simulink model "TrailerSoftware"  (R2019b)
settings: Solver=FixedStepDiscrete  StartTime=0.0  StopTime=inf  FixedStep=update  RelTol=1e-3  EnableMultiTasking=on
values from neighbouring files (symbols this model uses):
  countmax1 = 2500    [ProductionMfile.m]
  countmax2 = 2500    [ProductionMfile.m]
  HeaterIntGain = .0008    (= 0.0008)    [ProductionMfile.m]
  HeatGain = 10    [ProductionMfile.m]
  Intll = 0    [ProductionMfile.m]
  MaxCondPressure = 350    [ProductionMfile.m]
  MinSP = 1    [ProductionMfile.m]
  PostGain100 = 0.0002    [ProductionMfile.m]
  PostGain150 = 0.0005    [ProductionMfile.m]
  PostGain200 = 0.0004    [ProductionMfile.m]
  PostGain300 = 0.0008    [ProductionMfile.m]
  PostInit150 = 12    [ProductionMfile.m]
  PostIntulC = 65    [ProductionMfile.m]
  PostPGain = 0    [ProductionMfile.m]
  PreGain100 = 0.0005    [ProductionMfile.m]
  PreGain150 = 0.0005    [ProductionMfile.m]
  PreGain200 = 0.0003    [ProductionMfile.m]
  PreGain300 = 0.0008    [ProductionMfile.m]
  PreInit150 = 30    [ProductionMfile.m]
  PreIntulC = 65    [ProductionMfile.m]
  PreIntulDH = 65    [ProductionMfile.m]
  PrePGain = 0    [ProductionMfile.m]
  SatPress = [10 20 30 40 50 60 70 80 90 100 110 120 130 140 150 160 170      180 190 200 210 220 230 240 250 260 270 280 290 300 310 320 330      340 350 360 370 380 390 400 410 420 430 440 450 460 470 480 490      500]    [ProductionMfile.m]
  SatTemp = [-29.497 -2.4046 15.401 29.047 40.267 49.88 58.338 65.922 72.819      79.159 85.037 90.526 95.68 100.55 105.16 109.54 113.73 117.73 121.57      125.26 128.82 132.25 135.56 138.77 141.88 144.89 147.82 150.67 153.44      156.15 158.78 161.35 163.85 166.3 168.7 171.04 173.33 175.58 177.77      179.93 182.04 184.11 186.14 188.14 190.09 192.01 193.9 195.75 197.58      199.37]    [ProductionMfile.m]
  SHGain = 2    [ProductionMfile.m]
  SizeCANMatrix = 80    [ProductionMfile.m]
  SizeCOBIDVector = 10    [ProductionMfile.m]
  update = 0.002    [ProductionMfile.m]
undefined symbols (not defined in the file or in its folder): DiscIntNeverNeededParam, PostDGain, PreDGain, Ratio100, Ratio150, Ratio200, Ratio300
libraries: simulink x60, c2837xDlib x35, xpcutilitieslib x24, c2802xlib x8, c280xlib x7, etargetslib x4, svdutilitieslib x2, c2000lib x1
(part 4 of 8)

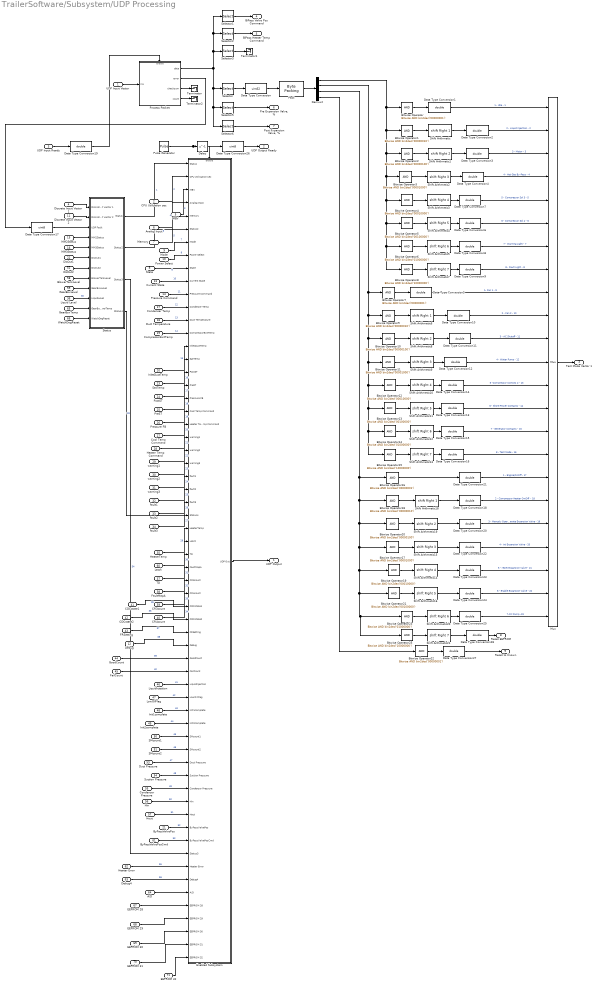
== system TrailerSoftware/Subsystem/UDP Processing ==
  UDP Input Vector : Inport  OutDataTypeStr=uint8  PortDimensions=SizeUDPInput  SampleTime=update  LockScale=on
  CPU Utilization sec : Inport  Port=2  OutDataTypeStr=double  PortDimensions=1  SampleTime=update
  UDP Input Ready : Inport  Port=3  OutDataTypeStr=boolean  PortDimensions=1  SampleTime=update
  Discrete Input Vector 1 : Inport  Port=4  OutDataTypeStr=uint8  PortDimensions=16  SampleTime=update
  MBV : Inport  Port=5  OutDataTypeStr=double  PortDimensions=MBVS  SampleTime=update
  Analog Input : Inport  Port=6
  Memory : Inport  Port=7
  State : Inport  Port=8
  Mode : Inport  Port=9
  Power Select : Inport  Port=10
  Discrete Input Vector 2 : Inport  Port=11  OutDataTypeStr=uint8  PortDimensions=16  SampleTime=update
  Debug : Inport  Port=12  PortDimensions=1
  Current State : Inport  Port=13  PortDimensions=1
  Pressure Command : Inport  Port=14
  MM2Status : Inport  Port=15
  MM3Status : Inport  Port=16  OutDataTypeStr=uint8  PortDimensions=1  SampleTime=update
  Condenser Temp : Inport  Port=17
  Duct Temperature : Inport  Port=18
  CompressorExitTemp : Inport  Port=19
  InletDuctTemp : Inport  Port=20
  ByPassValvePos : Inport  Port=21  OutDataTypeStr=double  SampleTime=update
  DisOut1 : Inport  Port=22  OutDataTypeStr=uint8  SampleTime=update
  SatTemp : Inport  Port=23
  PostST : Inport  Port=24
  PreST : Inport  Port=25
  Pressure FB : Inport  Port=26
  Cool Temp Command : Inport  Port=27
  Heater Temp Command : Inport  Port=28
  warning1 : Inport  Port=29
  warning2 : Inport  Port=30
  warning3 : Inport  Port=31
  fault1 : Inport  Port=32
  fault2 : Inport  Port=33
  fault3 : Inport  Port=34
  HeaterTemp : Inport  Port=35
  Liquid Level : Inport  Port=36
  TD : Inport  Port=37
  FaultMapA : Inport  Port=38
  CR3count : Inport  Port=39
  CR4count : Inport  Port=40
  CDCstate1 : Inport  Port=41
  CDCstate2 : Inport  Port=42
  FRSetting : Inport  Port=43
  GoodCount : Inport  Port=44  PortDimensions=1
  FailCount : Inport  Port=45  PortDimensions=1
  LiquidInjection : Inport  Port=46  PortDimensions=1
  LowOilFlag : Inport  Port=47
  Init1complete : Inport  Port=48  PortDimensions=1
  Init2complete : Inport  Port=49  PortDimensions=1
  SMcount1 : Inport  Port=50  PortDimensions=1
  SMcount2 : Inport  Port=51  PortDimensions=1
  DisOut2 : Inport  Port=52  OutDataTypeStr=uint8  SampleTime=update
  Duct Pressure : Inport  Port=53
  Suction Pressure : Inport  Port=54
  Condensor Pressure : Inport  Port=55
  Hin : Inport  Port=56
  Hout : Inport  Port=57
  BlowerTankLevel : Inport  Port=58
  GearBoxLevel : Inport  Port=59
  Latch : Inport  Port=60
  ByPassValvePosCmd : Inport  Port=61  OutDataTypeStr=double  SampleTime=update
  Heater Error : Inport  Port=62  PortDimensions=1
  Debug4 : Inport  Port=63  PortDimensions=1
  A/D : Inport  Port=64  PortDimensions=8
  GearBoxTemp : Inport  Port=65
  WatchDogReset : Inport  Port=66  OutDataTypeStr=uint8  PortDimensions=1  SampleTime=update
  EEPROM 28 : Inport  Port=67
  EEPROM 29 : Inport  Port=68
  EEPROM 30 : Inport  Port=69
  EEPROM 31 : Inport  Port=70
  EEPROM 32 : Inport  Port=71
  Bitwise Operator{,7,16,22} (4 alike) : simulink/Logic and Bit Operations/Bitwise Operator  logicop=AND  UseBitMask=on  BitMask=bin2dec('00000001')  BitMaskRealWorld=Stored Integer
  Bitwise Operator1 : simulink/Logic and Bit Operations/Bitwise Operator  logicop=AND  UseBitMask=on  BitMask=bin2dec('00000010')  BitMaskRealWorld=Stored Integer
  Bitwise Operator10 : simulink/Logic and Bit Operations/Bitwise Operator  logicop=AND  UseBitMask=on  BitMask=bin2dec('00000100')  BitMaskRealWorld=Stored Integer
  Bitwise Operator11 : simulink/Logic and Bit Operations/Bitwise Operator  logicop=AND  UseBitMask=on  BitMask=bin2dec('00001000')  BitMaskRealWorld=Stored Integer
  Bitwise Operator12 : simulink/Logic and Bit Operations/Bitwise Operator  logicop=AND  UseBitMask=on  BitMask=bin2dec('00010000')  BitMaskRealWorld=Stored Integer
  Bitwise Operator13 : simulink/Logic and Bit Operations/Bitwise Operator  logicop=AND  UseBitMask=on  BitMask=bin2dec('00100000')  BitMaskRealWorld=Stored Integer
  Bitwise Operator14 : simulink/Logic and Bit Operations/Bitwise Operator  logicop=AND  UseBitMask=on  BitMask=bin2dec('01000000')  BitMaskRealWorld=Stored Integer
  Bitwise Operator15 : simulink/Logic and Bit Operations/Bitwise Operator  logicop=AND  UseBitMask=on  BitMask=bin2dec('10000000')  BitMaskRealWorld=Stored Integer
  Bitwise Operator17 : simulink/Logic and Bit Operations/Bitwise Operator  logicop=AND  UseBitMask=on  BitMask=bin2dec('00001000')  BitMaskRealWorld=Stored Integer
  Bitwise Operator18 : simulink/Logic and Bit Operations/Bitwise Operator  logicop=AND  UseBitMask=on  BitMask=bin2dec('00000010')  BitMaskRealWorld=Stored Integer
  Bitwise Operator19 : simulink/Logic and Bit Operations/Bitwise Operator  logicop=AND  UseBitMask=on  BitMask=bin2dec('00010000')  BitMaskRealWorld=Stored Integer
  Bitwise Operator2 : simulink/Logic and Bit Operations/Bitwise Operator  logicop=AND  UseBitMask=on  BitMask=bin2dec('00000100')  BitMaskRealWorld=Stored Integer
  Bitwise Operator20 : simulink/Logic and Bit Operations/Bitwise Operator  logicop=AND  UseBitMask=on  BitMask=bin2dec('00000100')  BitMaskRealWorld=Stored Integer
  Bitwise Operator21 : simulink/Logic and Bit Operations/Bitwise Operator  logicop=AND  UseBitMask=on  BitMask=bin2dec('00100000')  BitMaskRealWorld=Stored Integer
  Bitwise Operator23 : simulink/Logic and Bit Operations/Bitwise Operator  logicop=AND  UseBitMask=on  BitMask=bin2dec('01000000')  BitMaskRealWorld=Stored Integer
  Bitwise Operator25 : simulink/Logic and Bit Operations/Bitwise Operator  logicop=AND  UseBitMask=on  BitMask=bin2dec('10000000')  BitMaskRealWorld=Stored Integer
  Bitwise Operator3 : simulink/Logic and Bit Operations/Bitwise Operator  logicop=AND  UseBitMask=on  BitMask=bin2dec('00001000')  BitMaskRealWorld=Stored Integer
  Bitwise Operator4 : simulink/Logic and Bit Operations/Bitwise Operator  logicop=AND  UseBitMask=on  BitMask=bin2dec('00010000')  BitMaskRealWorld=Stored Integer
  Bitwise Operator5 : simulink/Logic and Bit Operations/Bitwise Operator  logicop=AND  UseBitMask=on  BitMask=bin2dec('00100000')  BitMaskRealWorld=Stored Integer
  Bitwise Operator6 : simulink/Logic and Bit Operations/Bitwise Operator  logicop=AND  UseBitMask=on  BitMask=bin2dec('01000000')  BitMaskRealWorld=Stored Integer
  Bitwise Operator8 : simulink/Logic and Bit Operations/Bitwise Operator  logicop=AND  UseBitMask=on  BitMask=bin2dec('10000000')  BitMaskRealWorld=Stored Integer
  Bitwise Operator9 : simulink/Logic and Bit Operations/Bitwise Operator  logicop=AND  UseBitMask=on  BitMask=bin2dec('00000010')  BitMaskRealWorld=Stored Integer
  Data Type Conversion : DataTypeConversion  OutDataTypeStr=uint32
  Data Type Conversion{1..16,18..25,27..28} (26 alike) : DataTypeConversion  OutDataTypeStr=double
  Data Type Conversion17 : DataTypeConversion  OutDataTypeStr=uint8
  Data Type Conversion26 : DataTypeConversion  OutDataTypeStr=uint8
  Delay : Delay  DelayLength=1  InitialCondition=0
  Demux2 : Demux
  Enabled Subsystem : Subsystem  TreatAsAtomicUnit=on
  Mux : Mux  Inputs=23
  Pack : xpcutilitieslib/Byte Packing   MaskPackedDataType=uint8  MaskUnpackedDataTypes={'uint32'}  MaskAlignment=1
  Process Packet : Subsystem
  Pulse Generator : DiscretePulseGenerator  Period=10  SampleTime=update
  Selector : Selector  InputPortWidth=ndmain  IndexOptions=Index vector (dialog)  Indices=[1]  OutputSizes=1
  Selector1 : Selector  InputPortWidth=ndmain  IndexOptions=Index vector (dialog)  Indices=[2]  OutputSizes=1
  Selector2 : Selector  InputPortWidth=ndmain  IndexOptions=Index vector (dialog)  Indices=[3]  OutputSizes=1
  Selector3 : Selector  InputPortWidth=ndmain  IndexOptions=Index vector (dialog)  Indices=[4]  OutputSizes=1
  Selector5 : Selector  InputPortWidth=ndmain  IndexOptions=Index vector (dialog)  Indices=[6]  OutputSizes=1
  Selector6 : Selector  InputPortWidth=ndmain  IndexOptions=Index vector (dialog)  Indices=[7]  OutputSizes=1
  Shift Arithmetic : ArithShift  BitShiftNumber=1  BitShiftDirection=Right
  Shift Arithmetic1 : ArithShift  BitShiftNumber=2  BitShiftDirection=Right
  Shift Arithmetic10 : ArithShift  BitShiftNumber=4  BitShiftDirection=Right
  Shift Arithmetic11 : ArithShift  BitShiftNumber=5  BitShiftDirection=Right
  Shift Arithmetic12 : ArithShift  BitShiftNumber=6  BitShiftDirection=Right
  Shift Arithmetic13 : ArithShift  BitShiftNumber=7  BitShiftDirection=Right
  Shift Arithmetic14 : ArithShift  BitShiftNumber=4  BitShiftDirection=Right
  Shift Arithmetic15 : ArithShift  BitShiftNumber=3  BitShiftDirection=Right
  Shift Arithmetic16 : ArithShift  BitShiftNumber=5  BitShiftDirection=Right
  Shift Arithmetic18 : ArithShift  BitShiftNumber=1  BitShiftDirection=Right
  Shift Arithmetic19 : ArithShift  BitShiftNumber=2  BitShiftDirection=Right
  Shift Arithmetic2 : ArithShift  BitShiftNumber=3  BitShiftDirection=Right
  Shift Arithmetic20 : ArithShift  BitShiftNumber=6  BitShiftDirection=Right
  Shift Arithmetic21 : ArithShift  BitShiftNumber=7  BitShiftDirection=Right
  Shift Arithmetic3 : ArithShift  BitShiftNumber=4  BitShiftDirection=Right
  Shift Arithmetic4 : ArithShift  BitShiftNumber=5  BitShiftDirection=Right
  Shift Arithmetic5 : ArithShift  BitShiftNumber=6  BitShiftDirection=Right
  Shift Arithmetic6 : ArithShift  BitShiftNumber=1  BitShiftDirection=Right
  Shift Arithmetic7 : ArithShift  BitShiftNumber=7  BitShiftDirection=Right
  Shift Arithmetic8 : ArithShift  BitShiftNumber=2  BitShiftDirection=Right
  Shift Arithmetic9 : ArithShift  BitShiftNumber=3  BitShiftDirection=Right
  Status : Subsystem
  Terminator : Terminator
  Terminator1 : Terminator
  Terminator2 : Terminator
  UDP Output : Outport  OutDataTypeStr=uint8  PortDimensions=376  VectorParamsAs1DForOutWhenUnconnected=off
  UDP Output Ready : Outport  Port=2  OutDataTypeStr=uint8  SampleTime=update  VectorParamsAs1DForOutWhenUnconnected=off  LockScale=on
  Test Mode Vector 1 : Outport  Port=3  VectorParamsAs1DForOutWhenUnconnected=off
  BiPass Valve Pos Command : Outport  Port=4  VectorParamsAs1DForOutWhenUnconnected=off
  BiPass Heater Temp Command : Outport  Port=5  VectorParamsAs1DForOutWhenUnconnected=off
  "Pre Expansion Valve, %" : Outport  Port=6  VectorParamsAs1DForOutWhenUnconnected=off
  "Post Expansion Valve, %" : Outport  Port=7  VectorParamsAs1DForOutWhenUnconnected=off
  Reset EEPROM : Outport  Port=8  VectorParamsAs1DForOutWhenUnconnected=off
  Reset to Known : Outport  Port=9  VectorParamsAs1DForOutWhenUnconnected=off
  wires:
  Process Packet/1(data) -> Selector3/1, Selector1/1, Selector2/1, Selector6/1, Selector5/1, Selector/1
  Process Packet/4(count) -> Terminator2/1
  Process Packet/3(checksum) -> Terminator/1
  UDP Input Vector/1 -> Process Packet/1(In1)
  Bitwise Operator/1 -> Data Type Conversion1/1
  Bitwise Operator1/1 -> Shift Arithmetic/1
  Bitwise Operator2/1 -> Shift Arithmetic1/1
  Bitwise Operator3/1 -> Shift Arithmetic2/1
  Data Type Conversion4/1 -> Mux/4  "4 - Hot Gas By-Pass - 4"
  Bitwise Operator5/1 -> Shift Arithmetic4/1
  Data Type Conversion6/1 -> Mux/6  "6 - Compressor Sol 4 - 6"
  Bitwise Operator4/1 -> Shift Arithmetic3/1
  Data Type Conversion7/1 -> Mux/5  "5 - Compressor Sol 3 - 5"
  Shift Arithmetic/1 -> Data Type Conversion2/1
  Shift Arithmetic1/1 -> Data Type Conversion3/1
  Shift Arithmetic2/1 -> Data Type Conversion4/1
  Shift Arithmetic3/1 -> Data Type Conversion7/1
  Shift Arithmetic4/1 -> Data Type Conversion6/1
  Bitwise Operator6/1 -> Shift Arithmetic5/1
  Data Type Conversion8/1 -> Mux/7  "7 - Warning Light - 7"
  Shift Arithmetic5/1 -> Data Type Conversion8/1
  Bitwise Operator8/1 -> Shift Arithmetic7/1
  Shift Arithmetic7/1 -> Data Type Conversion9/1
  Data Type Conversion9/1 -> Mux/8  "8 - Fault Light - 8"
  Data Type Conversion1/1 -> Mux/1  "1 - Idle - 1"
  Data Type Conversion2/1 -> Mux/2  "2 - Liquid Injection - 2"
  Data Type Conversion3/1 -> Mux/3  "3 - Motor - 3"
  Demux2/1 -> Bitwise Operator/1, Bitwise Operator1/1, Bitwise Operator2/1, Bitwise Operator8/1, Bitwise Operator6/1, Bitwise Operator5/1, Bitwise Operator4/1, Bitwise Operator3/1
  Data Type Conversion/1 -> Pack/1
  Pack/1 -> Demux2/1
  Discrete Input Vector 1/1 -> Status/1(Discrete Input Vector 1)
  Status/1("Status ") -> Enabled Subsystem/1(Status)  "1"
  Bitwise Operator7/1 -> Data Type Conversion5/1
  Bitwise Operator9/1 -> Shift Arithmetic6/1
  Bitwise Operator10/1 -> Shift Arithmetic8/1
  Bitwise Operator11/1 -> Shift Arithmetic9/1
  Data Type Conversion12/1 -> Mux/12  "4 - Water Pump - 12"
  Bitwise Operator13/1 -> Shift Arithmetic11/1
  Data Type Conversion13/1 -> Mux/14  "6 - Shore Power Contacts - 14"
  Bitwise Operator12/1 -> Shift Arithmetic10/1
  Data Type Conversion14/1 -> Mux/13  "5 -Compressor Contcts 2 - 13"
  Shift Arithmetic6/1 -> Data Type Conversion10/1
  Shift Arithmetic8/1 -> Data Type Conversion11/1
  Shift Arithmetic9/1 -> Data Type Conversion12/1
  Shift Arithmetic10/1 -> Data Type Conversion14/1
  Shift Arithmetic11/1 -> Data Type Conversion13/1
  Bitwise Operator14/1 -> Shift Arithmetic12/1
  Data Type Conversion15/1 -> Mux/15  "7 - Generator Contacts - 15"
  Shift Arithmetic12/1 -> Data Type Conversion15/1
  Bitwise Operator15/1 -> Shift Arithmetic13/1
  Shift Arithmetic13/1 -> Data Type Conversion16/1
  Data Type Conversion16/1 -> Mux/16  "8 - Test Mode - 16"
  Data Type Conversion10/1 -> Mux/10  "2 - Fan 2 - 10"
  Data Type Conversion11/1 -> Mux/11  "3 - AC Shutoff - 11"
  Demux2/2 -> Bitwise Operator15/1, Bitwise Operator14/1, Bitwise Operator13/1, Bitwise Operator12/1, Bitwise Operator11/1, Bitwise Operator10/1, Bitwise Operator9/1, Bitwise Operator7/1
  Delay/1 -> Data Type Conversion26/1
  Mux/1 -> Test Mode Vector 1/1
  Data Type Conversion5/1 -> Mux/9  "1- Fan 1 - 9"
  CPU Utilization sec/1 -> Enabled Subsystem/2(CPU Utilization sec)  "2"
  MBV/1 -> Enabled Subsystem/3(MBV)  "3"
  Analog Input/1 -> Enabled Subsystem/4(Analog Input)  "4"
  Memory/1 -> Enabled Subsystem/5(Memory)  "5"
  State/1 -> Enabled Subsystem/9(State)  "9"
  Enabled Subsystem/1(UDP Out) -> UDP Output/1
  Mode/1 -> Enabled Subsystem/7(Mode)  "7"
  Power Select/1 -> Enabled Subsystem/8(Power Select)  "8"
  Discrete Input Vector 2/1 -> Status/2(Discrete Input Vector 2)
  Process Packet/2(error) -> Data Type Conversion17/1
  Data Type Conversion17/1 -> Status/3(UDP Fault)
  Current State/1 -> Enabled Subsystem/10(Current State)  "10"
  Pressure Command/1 -> Enabled Subsystem/11(Pressure Command)  "11"
  Selector5/1 -> "Pre Expansion Valve, %"/1
  Selector6/1 -> "Post Expansion Valve, %"/1
  MM3Status/1 -> Status/5(MM3Status)
  MM2Status/1 -> Status/4(MM2Status)
  Condenser Temp/1 -> Enabled Subsystem/12(Condenser Temp)  "12"
  Duct Temperature/1 -> Enabled Subsystem/13(Duct Temperature)  "13"
  CompressorExitTemp/1 -> Enabled Subsystem/14(CompressorExitTemp)  "14"
  Bitwise Operator16/1 -> Data Type Conversion21/1
  Data Type Conversion20/1 -> Mux/19  "3 - Manualy Opererate Expansion Valve - 19"
  Data Type Conversion21/1 -> Mux/17  "1 - Engine/OnOff - 17"
  Selector1/1 -> BiPass Valve Pos Command/1
  Selector2/1 -> BiPass Heater Temp Command/1
  Selector3/1 -> Terminator1/1
  InletDuctTemp/1 -> Enabled Subsystem/15(InletDuctTemp)  "15"
  ByPassValvePos/1 -> Enabled Subsystem/52(ByPassValvePos)  "52"
  DisOut1/1 -> Status/6(DisOut1)
  SatTemp/1 -> Enabled Subsystem/16(SatTemp)  "16"
  PostST/1 -> Enabled Subsystem/17(PostST)  "17"
  PreST/1 -> Enabled Subsystem/18(PreST)  "18"
  Pressure FB/1 -> Enabled Subsystem/19(Pressure FB)  "19"
  Cool Temp Command/1 -> Enabled Subsystem/20(Cool Temp Command)  "20"
  Heater Temp Command/1 -> Enabled Subsystem/21(Heater Temp Command)  "21"
  warning1/1 -> Enabled Subsystem/22(warning1)  "22"
  warning3/1 -> Enabled Subsystem/24(warning3)  "24"
  warning2/1 -> Enabled Subsystem/23(warning2)  "23"
  fault1/1 -> Enabled Subsystem/25(fault1)  "25"
  fault2/1 -> Enabled Subsystem/26(fault2)  "26"
  fault3/1 -> Enabled Subsystem/27(fault3)  "27"
  HeaterTemp/1 -> Enabled Subsystem/29(HeaterTemp)  "29"
  Latch/1 -> Enabled Subsystem/30(Latch)  "30"
  TD/1 -> Enabled Subsystem/31(TD)  "31"
  FaultMapA/1 -> Enabled Subsystem/32(FaultMapA)  "32"
  CR3count/1 -> Enabled Subsystem/33(CR3count)  "33"
  CR4count/1 -> Enabled Subsystem/34(CR4count)  "34"
  CDCstate1/1 -> Enabled Subsystem/35(CDCstate1)  "35"
  CDCstate2/1 -> Enabled Subsystem/36(CDCstate2)  "36"
  Debug/1 -> Enabled Subsystem/38(Debug)  "38"
  Status/2(Status2) -> Enabled Subsystem/6(Status2)  "6"
  FRSetting/1 -> Enabled Subsystem/37(FRSetting)  "37"
  Shift Arithmetic18/1 -> Data Type Conversion18/1
  Data Type Conversion18/1 -> Mux/18  "2 - Compressor Heater On/Off  - 18"
  GoodCount/1 -> Enabled Subsystem/39(GoodCount)  "39"
  FailCount/1 -> Enabled Subsystem/40(FailCount)  "40"
  LiquidInjection/1 -> Enabled Subsystem/41(LiquidInjection)  "41"
  LowOilFlag/1 -> Enabled Subsystem/42(LowOilFlag)  "42"
  Data Type Conversion22/1 -> Mux/20  "4 - int Expansion Valve - 20"
  Data Type Conversion23/1 -> Mux/21  "5 - reset Expansion Valve - 21"
  SMcount1/1 -> Enabled Subsystem/45(SMcount1)  "45"
  Init2complete/1 -> Enabled Subsystem/44(Init2complete)  "44"
  Init1complete/1 -> Enabled Subsystem/43(Init1complete)  "43"
  SMcount2/1 -> Enabled Subsystem/46(SMcount2)  "46"
  Status/4(Status4) -> Enabled Subsystem/28(Status4)  "28"
  Selector/1 -> Data Type Conversion/1
  Bitwise Operator18/1 -> Shift Arithmetic18/1
  Bitwise Operator20/1 -> Shift Arithmetic19/1
  Shift Arithmetic19/1 -> Data Type Conversion20/1
  Bitwise Operator17/1 -> Shift Arithmetic15/1
  Shift Arithmetic15/1 -> Data Type Conversion22/1
  Bitwise Operator19/1 -> Shift Arithmetic14/1
  Shift Arithmetic14/1 -> Data Type Conversion23/1
  Bitwise Operator21/1 -> Shift Arithmetic16/1
  Shift Arithmetic16/1 -> Data Type Conversion24/1
  Data Type Conversion24/1 -> Mux/22  "6 - Enable Expansion Valve - 22"
  DisOut2/1 -> Status/7(DisOut2)
  Bitwise Operator23/1 -> Shift Arithmetic20/1
  Shift Arithmetic20/1 -> Data Type Conversion25/1
  Data Type Conversion25/1 -> Mux/23  "7-Oil Pump -23"
  Duct Pressure/1 -> Enabled Subsystem/47(Duct Pressure)  "47"
  Suction Pressure/1 -> Enabled Subsystem/48(Suction Pressure)  "48"
  Condensor Pressure/1 -> Enabled Subsystem/49(Condensor Pressure)  "49"
  Hout/1 -> Enabled Subsystem/51(Hout)  "51"
  Hin/1 -> Enabled Subsystem/50(Hin)  "50"
  Data Type Conversion26/1 -> UDP Output Ready/1
  BlowerTankLevel/1 -> Status/8(BlowerTankLevel)
  GearBoxLevel/1 -> Status/9(GearBoxLevel)
  UDP Input Ready/1 -> Data Type Conversion19/1
  Liquid Level/1 -> Status/10(LiquidLevel)  "30"
  Pulse Generator/1 -> Enabled Subsystem/Enable, Delay/1
  Data Type Conversion19/1 -> Process Packet/Enable
  ByPassValvePosCmd/1 -> Enabled Subsystem/53(ByPassValvePosCmd)  "53"
  Status/3(Status3) -> Enabled Subsystem/54(Status3)  "54"
  Heater Error/1 -> Enabled Subsystem/55(Heater Error)  "55"
  Debug4/1 -> Enabled Subsystem/56(Debug4)  "56"
  A/D/1 -> Enabled Subsystem/57(A/D)
  GearBoxTemp/1 -> Status/11(GearBox OverTemp)
  WatchDogReset/1 -> Status/12(WatchDogReset)
  Data Type Conversion27/1 -> Reset to Known/1
  Bitwise Operator22/1 -> Data Type Conversion27/1
  Demux2/4 -> Bitwise Operator22/1
  Shift Arithmetic21/1 -> Data Type Conversion28/1
  Data Type Conversion28/1 -> Reset EEPROM/1
  EEPROM 28/1 -> Enabled Subsystem/58(EEPROM 28)
  EEPROM 29/1 -> Enabled Subsystem/59(EEPROM 29)
  EEPROM 30/1 -> Enabled Subsystem/60(EEPROM 30)
  EEPROM 31/1 -> Enabled Subsystem/61(EEPROM 31)
  EEPROM 32/1 -> Enabled Subsystem/62(EEPROM 32)
  Demux2/3 -> Bitwise Operator16/1, Bitwise Operator18/1, Bitwise Operator25/1, Bitwise Operator23/1, Bitwise Operator21/1, Bitwise Operator19/1, Bitwise Operator17/1, Bitwise Operator20/1
  Bitwise Operator25/1 -> Shift Arithmetic21/1

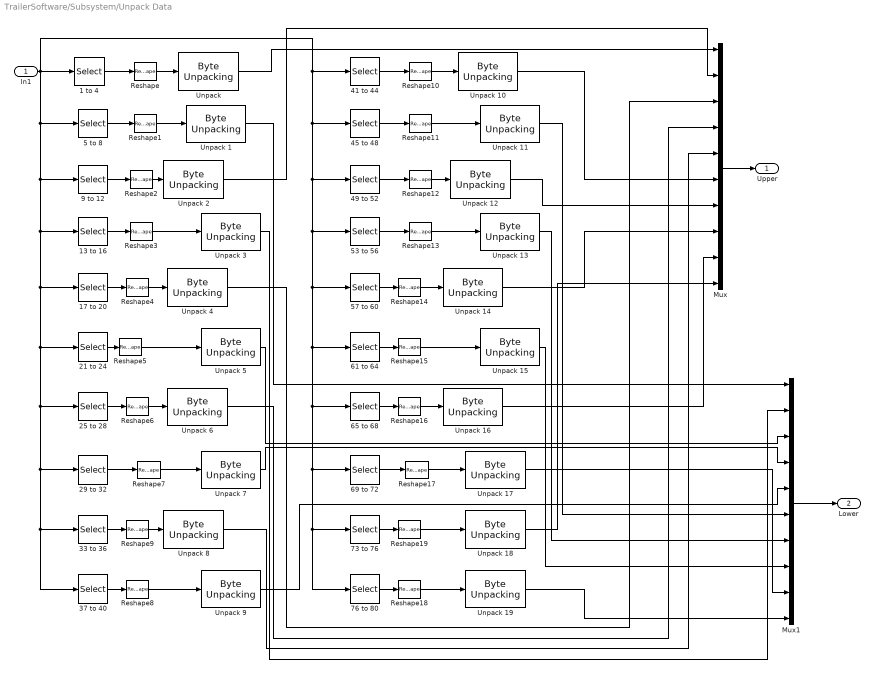
== system TrailerSoftware/Subsystem/Unpack Data ==
  In1 : Inport
  1 to 4 : Selector  InputPortWidth=80  IndexOptions=Index vector (dialog)  Indices=[1:4]  OutputSizes=1
  13 to 16 : Selector  InputPortWidth=80  IndexOptions=Index vector (dialog)  Indices=[13:16]  OutputSizes=1
  17 to 20 : Selector  InputPortWidth=80  IndexOptions=Index vector (dialog)  Indices=[17:20]  OutputSizes=1
  21 to 24 : Selector  InputPortWidth=80  IndexOptions=Index vector (dialog)  Indices=[21:24]  OutputSizes=1
  25 to 28 : Selector  InputPortWidth=80  IndexOptions=Index vector (dialog)  Indices=[25:28]  OutputSizes=1
  29 to 32 : Selector  InputPortWidth=80  IndexOptions=Index vector (dialog)  Indices=[29:32]  OutputSizes=1
  33 to 36 : Selector  InputPortWidth=80  IndexOptions=Index vector (dialog)  Indices=[33:36]  OutputSizes=1
  37 to 40 : Selector  InputPortWidth=80  IndexOptions=Index vector (dialog)  Indices=[37:40]  OutputSizes=1
  41 to 44 : Selector  InputPortWidth=80  IndexOptions=Index vector (dialog)  Indices=[41:44]  OutputSizes=1
  45 to 48 : Selector  InputPortWidth=80  IndexOptions=Index vector (dialog)  Indices=[45:48]  OutputSizes=1
  49 to 52 : Selector  InputPortWidth=80  IndexOptions=Index vector (dialog)  Indices=[49:52]  OutputSizes=1
  5 to 8 : Selector  InputPortWidth=80  IndexOptions=Index vector (dialog)  Indices=[5:8]  OutputSizes=1
  53 to 56 : Selector  InputPortWidth=80  IndexOptions=Index vector (dialog)  Indices=[53:56]  OutputSizes=1
  57 to 60 : Selector  InputPortWidth=80  IndexOptions=Index vector (dialog)  Indices=[57:60]  OutputSizes=1
  61 to 64 : Selector  InputPortWidth=80  IndexOptions=Index vector (dialog)  Indices=[61:64]  OutputSizes=1
  65 to 68 : Selector  InputPortWidth=80  IndexOptions=Index vector (dialog)  Indices=[65:68]  OutputSizes=1
  69 to 72 : Selector  InputPortWidth=80  IndexOptions=Index vector (dialog)  Indices=[69:72]  OutputSizes=1
  73 to 76 : Selector  InputPortWidth=80  IndexOptions=Index vector (dialog)  Indices=[73:76]  OutputSizes=1
  76 to 80 : Selector  InputPortWidth=80  IndexOptions=Index vector (dialog)  Indices=[77:80]  OutputSizes=1
  9 to 12 : Selector  InputPortWidth=80  IndexOptions=Index vector (dialog)  Indices=[9:12]  OutputSizes=1
  Mux : Mux  Inputs=10
  Mux1 : Mux  Inputs=10
  Reshape{,1..19} (20 alike) : Reshape
  Unpack {,1..19} (20 alike) : xpcutilitieslib/Byte Unpacking   MaskUnpackedDataTypes={'uint32'}  MaskUnpackedDataSizes={[1]}  MaskAlignment=1
      settings: SourceProductName=Simulink Real-Time  SourceProductBaseCode=XP
  Upper : Outport  VectorParamsAs1DForOutWhenUnconnected=off
  Lower : Outport  Port=2  VectorParamsAs1DForOutWhenUnconnected=off
  wires:
  1 to 4/1 -> Reshape/1
  5 to 8/1 -> Reshape1/1
  9 to 12/1 -> Reshape2/1
  13 to 16/1 -> Reshape3/1
  17 to 20/1 -> Reshape4/1
  21 to 24/1 -> Reshape5/1
  25 to 28/1 -> Reshape6/1
  29 to 32/1 -> Reshape7/1
  33 to 36/1 -> Reshape9/1
  37 to 40/1 -> Reshape8/1
  41 to 44/1 -> Reshape10/1
  45 to 48/1 -> Reshape11/1
  49 to 52/1 -> Reshape12/1
  53 to 56/1 -> Reshape13/1
  57 to 60/1 -> Reshape14/1
  61 to 64/1 -> Reshape15/1
  65 to 68/1 -> Reshape16/1
  69 to 72/1 -> Reshape17/1
  73 to 76/1 -> Reshape19/1
  76 to 80/1 -> Reshape18/1
  In1/1 -> 37 to 40/1, 33 to 36/1, 29 to 32/1, 25 to 28/1, 21 to 24/1, 17 to 20/1, 13 to 16/1, 9 to 12/1, 5 to 8/1, 76 to 80/1, 73 to 76/1, 69 to 72/1, 65 to 68/1, 61 to 64/1, 57 to 60/1, 53 to 56/1, 49 to 52/1, 45 to 48/1, 41 to 44/1, 1 to 4/1
  "Unpack "/1 -> Mux/1
  Unpack 2/1 -> Mux/2
  Unpack 4/1 -> Mux/3
  Unpack 6/1 -> Mux/4
  Unpack 8/1 -> Mux/5
  Unpack 10/1 -> Mux/6
  Unpack 12/1 -> Mux/7
  Unpack 14/1 -> Mux/8
  Unpack 16/1 -> Mux/9
  Unpack 18/1 -> Mux/10
  Mux/1 -> Upper/1
  Mux1/1 -> Lower/1
  Unpack 1/1 -> Mux1/1
  Unpack 3/1 -> Mux1/2
  Unpack 5/1 -> Mux1/3
  Unpack 7/1 -> Mux1/4
  Unpack 9/1 -> Mux1/5
  Unpack 11/1 -> Mux1/6
  Unpack 13/1 -> Mux1/7
  Unpack 15/1 -> Mux1/8
  Unpack 17/1 -> Mux1/9
  Unpack 19/1 -> Mux1/10
  Reshape/1 -> "Unpack "/1
  Reshape1/1 -> Unpack 1/1
  Reshape2/1 -> Unpack 2/1
  Reshape3/1 -> Unpack 3/1
  Reshape4/1 -> Unpack 4/1
  Reshape5/1 -> Unpack 5/1
  Reshape6/1 -> Unpack 6/1
  Reshape7/1 -> Unpack 7/1
  Reshape8/1 -> Unpack 9/1
  Reshape9/1 -> Unpack 8/1
  Reshape10/1 -> Unpack 10/1
  Reshape11/1 -> Unpack 11/1
  Reshape12/1 -> Unpack 12/1
  Reshape13/1 -> Unpack 13/1
  Reshape14/1 -> Unpack 14/1
  Reshape15/1 -> Unpack 15/1
  Reshape16/1 -> Unpack 16/1
  Reshape17/1 -> Unpack 17/1
  Reshape18/1 -> Unpack 19/1
  Reshape19/1 -> Unpack 18/1

== system TrailerSoftware/Subsystem/Super Heat Control/filter ==
  In1 : Inport
  Discrete-Time Integrator : DiscreteIntegrator  SampleTime=update  ICPrevOutput=DiscIntNeverNeededParam  ICPrevScaledInput=DiscIntNeverNeededParam
  K : Gain  Gain=.25
  Quantizer : Quantizer  QuantizationInterval=.5
  Saturation : Saturate  UpperLimit=3  LowerLimit=-3
  Sum2 : Sum  Inputs=|+-
  Out1 : Outport  VectorParamsAs1DForOutWhenUnconnected=off
  wires:
  Saturation/1 -> Discrete-Time Integrator/1
  In1/1 -> Sum2/1
  Sum2/1 -> K/1
  K/1 -> Saturation/1
  Discrete-Time Integrator/1 -> Sum2/2, Quantizer/1
  Quantizer/1 -> Out1/1

== system TrailerSoftware/Subsystem/Super Heat Control/filter1 ==
  In1 : Inport
  Discrete-Time Integrator : DiscreteIntegrator  SampleTime=update  ICPrevOutput=DiscIntNeverNeededParam  ICPrevScaledInput=DiscIntNeverNeededParam
  K : Gain  Gain=.25
  Quantizer : Quantizer  QuantizationInterval=.5
  Saturation : Saturate  UpperLimit=3  LowerLimit=-3
  Sum2 : Sum  Inputs=|+-
  Out1 : Outport  VectorParamsAs1DForOutWhenUnconnected=off
  wires:
  Saturation/1 -> Discrete-Time Integrator/1
  In1/1 -> Sum2/1
  Sum2/1 -> K/1
  K/1 -> Saturation/1
  Discrete-Time Integrator/1 -> Sum2/2, Quantizer/1
  Quantizer/1 -> Out1/1

== system TrailerSoftware/Subsystem/Super Heat Control/filter2 ==
  In1 : Inport
  Discrete-Time Integrator : DiscreteIntegrator  InitialCondition=70  SampleTime=update  ICPrevOutput=DiscIntNeverNeededParam  ICPrevScaledInput=DiscIntNeverNeededParam
  K : Gain  Gain=.05
  Quantizer : Quantizer  QuantizationInterval=10
  Saturation : Saturate  UpperLimit=3  LowerLimit=-3
  Sum2 : Sum  Inputs=|+-
  Out1 : Outport  VectorParamsAs1DForOutWhenUnconnected=off
  wires:
  Saturation/1 -> Discrete-Time Integrator/1
  In1/1 -> Sum2/1
  Sum2/1 -> K/1
  K/1 -> Saturation/1
  Discrete-Time Integrator/1 -> Sum2/2, Quantizer/1
  Quantizer/1 -> Out1/1

== system TrailerSoftware/Subsystem/Temperature Vector/DegCtoDegF ==
  In1 : Inport
  Constant7 : Constant  Value=32
  Gain9 : Gain  Gain=9/5
  Sum8 : Sum  Inputs=|++
  Out1 : Outport  VectorParamsAs1DForOutWhenUnconnected=off
  wires:
  Sum8/1 -> Out1/1
  In1/1 -> Gain9/1
  Constant7/1 -> Sum8/2
  Gain9/1 -> Sum8/1

== system TrailerSoftware/Subsystem/Temperature Vector/DegCtoDegF1 ==
  In1 : Inport
  Constant7 : Constant  Value=32
  Gain9 : Gain  Gain=9/5
  Sum8 : Sum  Inputs=|++
  Out1 : Outport  VectorParamsAs1DForOutWhenUnconnected=off
  wires:
  Sum8/1 -> Out1/1
  In1/1 -> Gain9/1
  Constant7/1 -> Sum8/2
  Gain9/1 -> Sum8/1

== system TrailerSoftware/Subsystem/Temperature Vector/DegCtoDegF2 ==
  In1 : Inport
  Constant7 : Constant  Value=32
  Gain9 : Gain  Gain=9/5
  Sum8 : Sum  Inputs=|++
  Out1 : Outport  VectorParamsAs1DForOutWhenUnconnected=off
  wires:
  Sum8/1 -> Out1/1
  In1/1 -> Gain9/1
  Constant7/1 -> Sum8/2
  Gain9/1 -> Sum8/1

== system TrailerSoftware/Subsystem/Temperature Vector/DegCtoDegF3 ==
  In1 : Inport
  Constant7 : Constant  Value=32
  Gain9 : Gain  Gain=9/5
  Sum8 : Sum  Inputs=|++
  Out1 : Outport  VectorParamsAs1DForOutWhenUnconnected=off
  wires:
  Sum8/1 -> Out1/1
  In1/1 -> Gain9/1
  Constant7/1 -> Sum8/2
  Gain9/1 -> Sum8/1

== system TrailerSoftware/Subsystem/Temperature Vector/DegCtoDegF4 ==
  In1 : Inport
  Constant7 : Constant  Value=32
  Gain9 : Gain  Gain=9/5
  Sum8 : Sum  Inputs=|++
  Out1 : Outport  VectorParamsAs1DForOutWhenUnconnected=off
  wires:
  Sum8/1 -> Out1/1
  In1/1 -> Gain9/1
  Constant7/1 -> Sum8/2
  Gain9/1 -> Sum8/1

== system TrailerSoftware/Subsystem/Temperature Vector/DegCtoDegF5 ==
  In1 : Inport
  Constant7 : Constant  Value=32
  Gain9 : Gain  Gain=9/5
  Sum8 : Sum  Inputs=|++
  Out1 : Outport  VectorParamsAs1DForOutWhenUnconnected=off
  wires:
  Sum8/1 -> Out1/1
  In1/1 -> Gain9/1
  Constant7/1 -> Sum8/2
  Gain9/1 -> Sum8/1

== system TrailerSoftware/Subsystem/Temperature Vector/DegCtoDegF6 ==
  In1 : Inport
  Constant7 : Constant  Value=32
  Gain9 : Gain  Gain=9/5
  Sum8 : Sum  Inputs=|++
  Out1 : Outport  VectorParamsAs1DForOutWhenUnconnected=off
  wires:
  Sum8/1 -> Out1/1
  In1/1 -> Gain9/1
  Constant7/1 -> Sum8/2
  Gain9/1 -> Sum8/1

== system TrailerSoftware/Subsystem/Temperature Vector/DegCtoDegF7 ==
  In1 : Inport
  Constant7 : Constant  Value=32
  Gain9 : Gain  Gain=9/5
  Sum8 : Sum  Inputs=|++
  Out1 : Outport  VectorParamsAs1DForOutWhenUnconnected=off
  wires:
  Sum8/1 -> Out1/1
  In1/1 -> Gain9/1
  Constant7/1 -> Sum8/2
  Gain9/1 -> Sum8/1

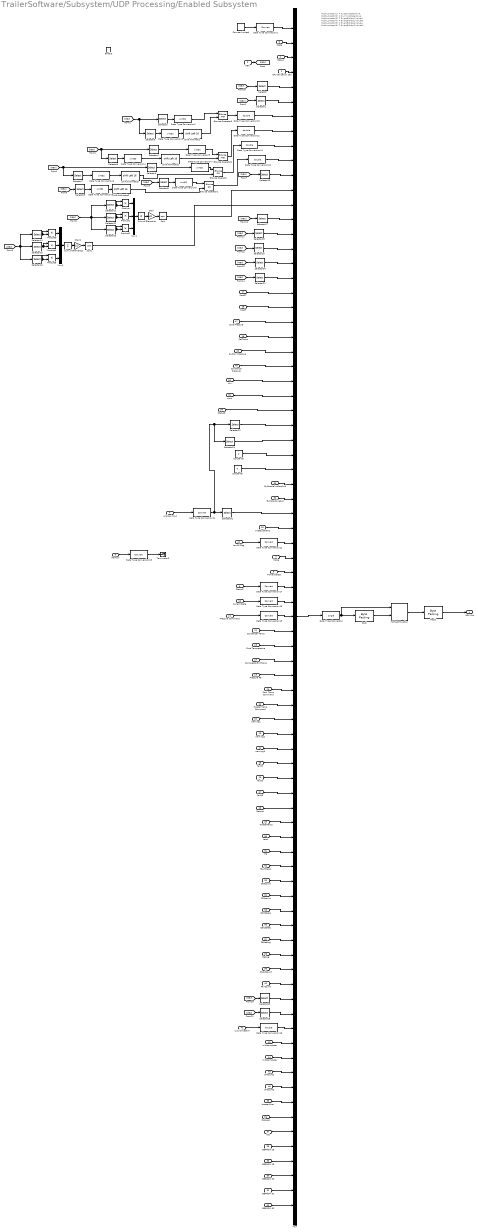
== system TrailerSoftware/Subsystem/UDP Processing/Enabled Subsystem ==
  note: ModbusVector(1) = SystemStateValue;
      | ModbusVector(2) = RunningStateValue;
      | ModbusVector(3) = EventBitMap1ValueA;
      | ModbusVector(4) = EventBitMap1ValueB;
      | ModbusVector(5) = EventBitMap2ValueA;
      | ModbusVector(6) = EventBitMap2ValueB;
      | ModbusVector(7) = FaultBitMapValueA;
      | ModbusVector(8) = FaultBitMapValueB;
      | ModbusVector(9) = WarningBitMapValueA;
      | ModbusVector(10) = WarningBitMapValueB;
      | ModbusVector(11) = GenFreqValue;
      | ModbusVector(12) = GenVoltValueA;
      | ModbusVector(13) = GenVoltValueB;
      | ModbusVector(14) = GenVoltValueC;
      | ModbusVector(15) = GenCurValueA;
      | ModbusVector(16) = GenCurValueB;
      | ModbusVector(17) = GenCurValueC;
      | ModbusVector(18) = EngineTempValue;
      | ModbusVector(19) = EngineOilPressValue;
      | ModbusVector(20) = FuelLevelValue;
      | ModbusVector(21) = BatteryVoltValue;
      | ModbusVector(22) = EngineRunHoursValue;
      | ModbusVector(23) = FCSuperHeatValue;
      | ModbusVector(24) = RCSuperHeatValue;
      | ModbusVector(25) = SuctionPressValue;
      | ModbusVector(26) = FSatTempValue;
      | ModbusVector(27) = RSatTempValue;
      | ModbusVector(28) = FSucTempValue;
      | ModbusVector(29) = RSucTempValue;
      | ModbusVector(30) = FRmTempValue;
      | ModbusVector(31) = RRmTempValue;
      | ModbusVector(32) = FValPosValue;
      | ModbusVector(33) = RValPosValue;
      | ModbusVector(34) = FEvapTempValue;
      | ModbusVector(35) = REvapTempValue;
      | ModbusVector(36) = FAlarmValue;
      | ModbusVector(37) = RAlarmValue;
  Status : Inport
  CPU Utilization sec : Inport  Port=2  OutDataTypeStr=double  PortDimensions=1  SampleTime=update
  MBV : Inport  Port=3  PortDimensions=MBVS
  Analog Input : Inport  Port=4
  Memory : Inport  Port=5
  Status2 : Inport  Port=6
  Mode : Inport  Port=7
  Power Select : Inport  Port=8
  State : Inport  Port=9
  Current State : Inport  Port=10
  Pressure Command : Inport  Port=11
  Condenser Temp : Inport  Port=12
  Duct Temperature : Inport  Port=13
  CompressorExitTemp : Inport  Port=14
  InletDuctTemp : Inport  Port=15
  SatTemp : Inport  Port=16
  PostST : Inport  Port=17
  PreST : Inport  Port=18
  Pressure FB : Inport  Port=19
  Cool Temp Command : Inport  Port=20
  Heater Temp Command : Inport  Port=21
  warning1 : Inport  Port=22
  warning2 : Inport  Port=23
  warning3 : Inport  Port=24
  fault1 : Inport  Port=25
  fault2 : Inport  Port=26
  fault3 : Inport  Port=27
  Status4 : Inport  Port=28
  HeaterTemp : Inport  Port=29
  Latch : Inport  Port=30
  TD : Inport  Port=31
  FaultMapA : Inport  Port=32
  CR3count : Inport  Port=33
  CR4count : Inport  Port=34
  CDCstate1 : Inport  Port=35
  CDCstate2 : Inport  Port=36
  FRSetting : Inport  Port=37
  Debug : Inport  Port=38  PortDimensions=1
  GoodCount : Inport  Port=39  PortDimensions=1
  FailCount : Inport  Port=40  PortDimensions=1
  LiquidInjection : Inport  Port=41  PortDimensions=1
  LowOilFlag : Inport  Port=42
  Init1complete : Inport  Port=43  PortDimensions=1
  Init2complete : Inport  Port=44  PortDimensions=1
  SMcount1 : Inport  Port=45  PortDimensions=1
  SMcount2 : Inport  Port=46  PortDimensions=1
  Duct Pressure : Inport  Port=47
  Suction Pressure : Inport  Port=48
  Condensor Pressure : Inport  Port=49
  Hin : Inport  Port=50
  Hout : Inport  Port=51
  ByPassValvePos : Inport  Port=52  OutDataTypeStr=double  SampleTime=update
  ByPassValvePosCmd : Inport  Port=53  OutDataTypeStr=double  SampleTime=update
  Status3 : Inport  Port=54
  Heater Error : Inport  Port=55  PortDimensions=1
  Debug4 : Inport  Port=56  PortDimensions=1
  A/D : Inport  Port=57  PortDimensions=8
  EEPROM 28 : Inport  Port=58
  EEPROM 29 : Inport  Port=59
  EEPROM 30 : Inport  Port=60
  EEPROM 31 : Inport  Port=61
  EEPROM 32 : Inport  Port=62
  Enable : EnablePort
  Bitwise Operator : simulink/Logic and Bit Operations/Bitwise Operator  logicop=OR  UseBitMask=off  NumInputPorts=2  BitMask=bin2dec('11011001')  BitMaskRealWorld=Stored Integer
  Bitwise Operator1 : simulink/Logic and Bit Operations/Bitwise Operator  logicop=OR  UseBitMask=off  NumInputPorts=2  BitMask=bin2dec('11011001')  BitMaskRealWorld=Stored Integer
  Bitwise Operator2 : simulink/Logic and Bit Operations/Bitwise Operator  logicop=AND  UseBitMask=off  NumInputPorts=2  BitMask=bin2dec('11011001')  BitMaskRealWorld=Stored Integer
  Bitwise Operator3 : simulink/Logic and Bit Operations/Bitwise Operator  logicop=AND  UseBitMask=off  NumInputPorts=2  BitMask=bin2dec('11011001')  BitMaskRealWorld=Stored Integer
  Constant8 : Constant  Value=0
  Constant9 : Constant  Value=0
  Counter Limited : simulink/Sources/Counter Limited  uplimit=2^30  tsamp=-1
  Data Type Conversion : DataTypeConversion  OutDataTypeStr=single
  Data Type Conversion{1,14..15,17..19,21} (7 alike) : DataTypeConversion
  Data Type Conversion{10..13,16} (5 alike) : DataTypeConversion  OutDataTypeStr=double
  Data Type Conversion{2..9} (8 alike) : DataTypeConversion  OutDataTypeStr=uint32
  Gain : Gain  Gain=1/3
  Gain1 : Gain  Gain=1/3
  MATLAB Function : MATLAB Function
  Mux : Mux  Inputs=81
  Mux1 : Mux  Inputs=3
  Mux2 : Mux  Inputs=3
  Pack : xpcutilitieslib/Byte Packing   MaskPackedDataType=uint8  MaskUnpackedDataTypes={'single'}  MaskAlignment=1
  Pack1 : xpcutilitieslib/Byte Packing   MaskPackedDataType=uint8  MaskUnpackedDataTypes={'single'}  MaskAlignment=4
  Product{,1..5} (6 alike) : Product
  Selector : Selector  InputPortWidth=MBVS  IndexOptions=Index vector (dialog)  Indices=[1]  OutputSizes=1
  Selector1 : Selector  InputPortWidth=MBVS  IndexOptions=Index vector (dialog)  Indices=[2]  OutputSizes=1
  Selector10 : Selector  IndexOptions=Index vector (dialog)  Indices=[11]  OutputSizes=1
  Selector11 : Selector  IndexOptions=Index vector (dialog)  Indices=[12]  OutputSizes=1
  Selector12 : Selector  IndexOptions=Index vector (dialog)  Indices=[13]  OutputSizes=1
  Selector13 : Selector  IndexOptions=Index vector (dialog)  Indices=[14]  OutputSizes=1
  Selector14 : Selector  IndexOptions=Index vector (dialog)  Indices=[15]  OutputSizes=1
  Selector15 : Selector  IndexOptions=Index vector (dialog)  Indices=[16]  OutputSizes=1
  Selector16 : Selector  IndexOptions=Index vector (dialog)  Indices=[17]  OutputSizes=1
  Selector17 : Selector  IndexOptions=Index vector (dialog)  Indices=[18]  OutputSizes=1
  Selector18 : Selector  IndexOptions=Index vector (dialog)  Indices=[19]  OutputSizes=1
  Selector19 : Selector  IndexOptions=Index vector (dialog)  Indices=[20]  OutputSizes=1
  Selector2 : Selector  IndexOptions=Index vector (dialog)  Indices=[3]  OutputSizes=1
  Selector20 : Selector  IndexOptions=Index vector (dialog)  Indices=[21]  OutputSizes=1
  Selector21 : Selector  IndexOptions=Index vector (dialog)  Indices=[22]  OutputSizes=1
  Selector22 : Selector  InputPortWidth=8  IndexOptions=Index vector (dialog)  Indices=[6]  OutputSizes=1
  Selector23 : Selector  IndexOptions=Index vector (dialog)  Indices=[38]  OutputSizes=1
  Selector24 : Selector  InputPortWidth=8  IndexOptions=Index vector (dialog)  Indices=[7]  OutputSizes=1
  Selector25 : Selector  IndexOptions=Index vector (dialog)  Indices=[39]  OutputSizes=1
  Selector3 : Selector  IndexOptions=Index vector (dialog)  Indices=[4]  OutputSizes=1
  Selector31 : Selector  InputPortWidth=8  IndexOptions=Index vector (dialog)  Indices=[1:6]  OutputSizes=1
  Selector4 : Selector  IndexOptions=Index vector (dialog)  Indices=[5]  OutputSizes=1
  Selector5 : Selector  IndexOptions=Index vector (dialog)  Indices=[6]  OutputSizes=1
  Selector6 : Selector  IndexOptions=Index vector (dialog)  Indices=[7]  OutputSizes=1
  Selector7 : Selector  IndexOptions=Index vector (dialog)  Indices=[8]  OutputSizes=1
  Selector8 : Selector  IndexOptions=Index vector (dialog)  Indices=[9]  OutputSizes=1
  Selector9 : Selector  IndexOptions=Index vector (dialog)  Indices=[10]  OutputSizes=1
  Shift Arithmetic{,1..3} (4 alike) : ArithShift  BitShiftNumber=16  BitShiftDirection=Left
  Sqrt : Sqrt  SaturateOnIntegerOverflow=on
  Sqrt1 : Sqrt  SaturateOnIntegerOverflow=on
  Sum of Elements : Sum  Inputs=+
  Sum of Elements1 : Sum  Inputs=+
  Terminator2 : Terminator
  UDP Out : Outport  PortDimensions=376  VectorParamsAs1DForOutWhenUnconnected=off
  wires:
  Counter Limited/1 -> Data Type Conversion1/1
  Data Type Conversion/1 -> MATLAB Function/1(u), Pack/1
  Pack/1 -> MATLAB Function/2(u2)
  MATLAB Function/1(y) -> Pack1/1
  Data Type Conversion1/1 -> Mux/1  "1"
  Status/1 -> Mux/3  "3"
  Selector/1 -> Mux/5  "5 - EG System State"
  Selector1/1 -> Mux/6  "6 - EG Running State"
  Data Type Conversion13/1 -> Mux/7  "7 - EG Event Bit Map 1"
  Bitwise Operator2/1 -> Data Type Conversion12/1
  Bitwise Operator/1 -> Data Type Conversion11/1
  CPU Utilization sec/1 -> Mux/4  "4"
  Mux/1 -> Data Type Conversion/1
  Selector2/1 -> Data Type Conversion2/1
  Selector3/1 -> Data Type Conversion3/1
  Data Type Conversion3/1 -> Shift Arithmetic/1
  Shift Arithmetic/1 -> Bitwise Operator3/2
  Data Type Conversion2/1 -> Bitwise Operator3/1
  Selector5/1 -> Data Type Conversion4/1
  Selector4/1 -> Data Type Conversion5/1
  Data Type Conversion4/1 -> Shift Arithmetic1/1
  Shift Arithmetic1/1 -> Bitwise Operator2/2
  Data Type Conversion5/1 -> Bitwise Operator2/1
  Selector7/1 -> Data Type Conversion6/1
  Selector6/1 -> Data Type Conversion7/1
  Data Type Conversion6/1 -> Shift Arithmetic3/1
  Shift Arithmetic3/1 -> Bitwise Operator/2
  Data Type Conversion7/1 -> Bitwise Operator/1
  Bitwise Operator1/1 -> Data Type Conversion10/1
  Selector9/1 -> Data Type Conversion8/1
  Selector8/1 -> Data Type Conversion9/1
  Data Type Conversion8/1 -> Shift Arithmetic2/1
  Shift Arithmetic2/1 -> Bitwise Operator1/2
  Data Type Conversion9/1 -> Bitwise Operator1/1
  Data Type Conversion10/1 -> Mux/10  "10 - EG Warning Bit Map"
  Data Type Conversion11/1 -> Mux/9  "9 - EG Fault Bit Map"
  Bitwise Operator3/1 -> Data Type Conversion13/1
  Selector10/1 -> Mux/11  "11 - Generator Frequency"
  Sqrt/1 -> Mux/12  "12 - RMS Voltage"
  Selector11/1 -> Product/2, Product/1
  Selector12/1 -> Product1/1, Product1/2
  Selector13/1 -> Product2/1, Product2/2
  Product2/1 -> Mux1/3
  Product1/1 -> Mux1/2
  Product/1 -> Mux1/1
  Mux1/1 -> Sum of Elements/1
  Sum of Elements/1 -> Gain/1
  Gain/1 -> Sqrt/1
  Sqrt1/1 -> Mux/13  "13 - RMS Current"
  Selector14/1 -> Product3/2, Product3/1
  Selector15/1 -> Product4/1, Product4/2
  Selector16/1 -> Product5/1, Product5/2
  Product5/1 -> Mux2/3
  Product4/1 -> Mux2/2
  Product3/1 -> Mux2/1
  Mux2/1 -> Sum of Elements1/1
  Sum of Elements1/1 -> Gain1/1
  Gain1/1 -> Sqrt1/1
  Selector17/1 -> Mux/14  "14 - Engine Temp Deg F"
  Selector18/1 -> Mux/15  "15 - Engine Oil Pressure, psi"
  Selector19/1 -> Mux/16  "16 - Fuel Level, %"
  Selector20/1 -> Mux/17  "17 - Battery Volts, volts"
  Selector21/1 -> Mux/18  "18 - Engine Run Hours"
  PostST/1 -> Mux/19  "19 - Post Super Heat Temperature, deg F"
  PreST/1 -> Mux/20  "20 -Pre Super Heat Temperature, deg F"
  Duct Pressure/1 -> Mux/21  "21 - Duct Pressure, psia"
  SatTemp/1 -> Mux/22  "22 -Saturation Temperature, deg F"
  Suction Pressure/1 -> Mux/23  "23"
  Condensor Pressure/1 -> Mux/24  "24 - Condensor Pressure"
  Hin/1 -> Mux/25  "25 - Hin"
  Hout/1 -> Mux/26  "26 - Hout"
  Status3/1 -> Mux/27  "27 - Status3"
  Selector22/1 -> Mux/28  "28 - Post Temperature"
  Selector24/1 -> Mux/29  "29 Pre Temperature"
  Constant8/1 -> Mux/30  "30 - Post Evaperature Out Temperature, deg F"
  Constant9/1 -> Mux/31  "31 - Pre Evaperature Out Temperature, deg F"
  Memory/1 -> Data Type Conversion15/1
  Data Type Conversion14/1 -> Selector24/1, Selector22/1, Selector31/1  "34-39"
  MBV/1 -> [MBV]
  [MBV] -> Selector/1
  [MBV] -> Selector1/1
  [MBV] -> Selector3/1, Selector2/1
  [MBV] -> Selector5/1, Selector4/1
  [MBV] -> Selector7/1, Selector6/1
  [MBV] -> Selector8/1
  [MBV] -> Selector9/1
  [MBV] -> Selector10/1
  [MBV] -> Selector13/1, Selector11/1, Selector12/1
  [MBV] -> Selector16/1, Selector14/1, Selector15/1
  [MBV] -> Selector17/1
  [MBV] -> Selector18/1
  [MBV] -> Selector19/1
  [MBV] -> Selector20/1
  [MBV] -> Selector21/1
  Analog Input/1 -> Data Type Conversion14/1
  Data Type Conversion15/1 -> Terminator2/1
  Status2/1 -> Data Type Conversion17/1
  Pack1/1 -> UDP Out/1
  Mode/1 -> Mux/37  "42"
  Power Select/1 -> Mux/38  "43"
  State/1 -> Mux/2  "2"
  Current State/1 -> Data Type Conversion18/1  "45"
  Pressure Command/1 -> Data Type Conversion19/1  "46"
  Condenser Temp/1 -> Mux/42  "47"
  Duct Temperature/1 -> Mux/43  "48"
  CompressorExitTemp/1 -> Mux/44  "49"
  Data Type Conversion17/1 -> Mux/39  "44"
  Data Type Conversion18/1 -> Mux/40
  Data Type Conversion19/1 -> Mux/41
  Selector31/1 -> Mux/34
  InletDuctTemp/1 -> Mux/35  "40"
  LowOilFlag/1 -> Data Type Conversion21/1  "41"
  Heater Temp Command/1 -> Mux/47  "52"
  Pressure FB/1 -> Mux/45  "50"
  Cool Temp Command/1 -> Mux/46  "51"
  warning1/1 -> Mux/48  "53"
  warning2/1 -> Mux/49  "54"
  warning3/1 -> Mux/50  "55"
  fault1/1 -> Mux/51  "56"
  fault2/1 -> Mux/52  "57"
  fault3/1 -> Mux/53  "58"
  Status4/1 -> Mux/54  "59 Status4"
  HeaterTemp/1 -> Mux/55  "60"
  Latch/1 -> Mux/56  "61"
  TD/1 -> Mux/57  "62"
  FaultMapA/1 -> Mux/58  "63"
  Data Type Conversion12/1 -> Mux/8  "8 - EG Event Bit Map 2"
  CR3count/1 -> Mux/59  "64"
  CR4count/1 -> Mux/60  "65"
  CDCstate2/1 -> Mux/62  "67"
  CDCstate1/1 -> Mux/61  "66"
  LiquidInjection/1 -> Data Type Conversion16/1  "74"
  FRSetting/1 -> Mux/63  "68"
  Debug/1 -> Mux/64  "69"
  GoodCount/1 -> Mux/65  "70"
  FailCount/1 -> Mux/66  "71"
  Selector23/1 -> Mux/67  "72"
  Selector25/1 -> Mux/68  "73"
  [MBV] -> Selector23/1
  [MBV] -> Selector25/1
  Data Type Conversion16/1 -> Mux/69
  Data Type Conversion21/1 -> Mux/36
  SMcount1/1 -> Mux/72  "77"
  Init2complete/1 -> Mux/71  "76"
  Init1complete/1 -> Mux/70  "75"
  SMcount2/1 -> Mux/73  "78"
  ByPassValvePos/1 -> Mux/33  "33"
  ByPassValvePosCmd/1 -> Mux/32  "32"
  Heater Error/1 -> Mux/74  "79"
  Debug4/1 -> Mux/75  "80"
  A/D/1 -> Mux/76
  EEPROM 29/1 -> Mux/78
  EEPROM 30/1 -> Mux/79
  EEPROM 31/1 -> Mux/80
  EEPROM 32/1 -> Mux/81
  EEPROM 28/1 -> Mux/77

== system TrailerSoftware/Subsystem/UDP Processing/Process Packet ==
  In1 : Inport
  Enable : EnablePort
  MATLAB Function : MATLAB Function
  Unpack : xpcutilitieslib/Byte Unpacking   MaskUnpackedDataTypes={'single'}  MaskUnpackedDataSizes={[ndmain+1]}  MaskAlignment=1
      settings: SourceProductName=Simulink Real-Time  SourceProductBaseCode=XP
  data : Outport  VectorParamsAs1DForOutWhenUnconnected=off
  error : Outport  Port=2  VectorParamsAs1DForOutWhenUnconnected=off
  checksum : Outport  Port=3  VectorParamsAs1DForOutWhenUnconnected=off
  count : Outport  Port=4  VectorParamsAs1DForOutWhenUnconnected=off
  wires:
  MATLAB Function/1(y) -> data/1
  MATLAB Function/2(error) -> error/1
  Unpack/1 -> MATLAB Function/1(u)
  MATLAB Function/3(checksum) -> checksum/1
  In1/1 -> MATLAB Function/2(u2), Unpack/1
  MATLAB Function/4(countout) -> count/1

== system TrailerSoftware/Subsystem/UDP Processing/Status ==
  Discrete Input Vector 1 : Inport  OutDataTypeStr=uint8  PortDimensions=DiscreteInputSize  SampleTime=update
  Discrete Input Vector 2 : Inport  Port=2  OutDataTypeStr=uint8  PortDimensions=16  SampleTime=update
  UDP Fault : Inport  Port=3  OutDataTypeStr=uint8  PortDimensions=1  SampleTime=update
  MM2Status : Inport  Port=4
  MM3Status : Inport  Port=5  OutDataTypeStr=uint8  PortDimensions=1  SampleTime=update
  DisOut1 : Inport  Port=6  OutDataTypeStr=uint8  SampleTime=update
  DisOut2 : Inport  Port=7  OutDataTypeStr=uint8  SampleTime=update
  BlowerTankLevel : Inport  Port=8
  GearBoxLevel : Inport  Port=9
  LiquidLevel : Inport  Port=10
  GearBox OverTemp : Inport  Port=11
  WatchDogReset : Inport  Port=12  OutDataTypeStr=uint8  PortDimensions=1  SampleTime=update
  Data Type Conversion{,3..5} (4 alike) : DataTypeConversion
  Data Type Conversion1 : DataTypeConversion  OutDataTypeStr=uint8
  Data Type Conversion2 : DataTypeConversion  OutDataTypeStr=uint8
  MATLAB Function : MATLAB Function  TreatAsAtomicUnit=on
  "Status " : Outport  VectorParamsAs1DForOutWhenUnconnected=off
  Status2 : Outport  Port=2  VectorParamsAs1DForOutWhenUnconnected=off
  Status3 : Outport  Port=3  VectorParamsAs1DForOutWhenUnconnected=off
  Status4 : Outport  Port=4  VectorParamsAs1DForOutWhenUnconnected=off
  wires:
  Discrete Input Vector 1/1 -> MATLAB Function/1(DisIn1)
  Discrete Input Vector 2/1 -> MATLAB Function/2(DisIn2)
  MATLAB Function/1(Status1) -> Data Type Conversion/1
  Data Type Conversion/1 -> "Status "/1
  UDP Fault/1 -> MATLAB Function/3(UDPFault)
  MM2Status/1 -> Data Type Conversion1/1
  MM3Status/1 -> Data Type Conversion2/1
  Data Type Conversion1/1 -> MATLAB Function/4(ManualMode2Status)
  Data Type Conversion2/1 -> MATLAB Function/5(ManualMode3Status)
  DisOut1/1 -> MATLAB Function/6(DisOut1)
  Data Type Conversion4/1 -> Status2/1
  MATLAB Function/2(Status2) -> Data Type Conversion4/1
  DisOut2/1 -> MATLAB Function/7(DisOut2)
  BlowerTankLevel/1 -> MATLAB Function/8(BlowerTankLevel)
  GearBoxLevel/1 -> MATLAB Function/9(GearBoxLevel)
  LiquidLevel/1 -> MATLAB Function/10(LiquidLevel)
  MATLAB Function/4(Status4) -> Data Type Conversion5/1
  MATLAB Function/3(Status3) -> Data Type Conversion3/1
  Data Type Conversion5/1 -> Status4/1
  Data Type Conversion3/1 -> Status3/1
  GearBox OverTemp/1 -> MATLAB Function/11(GearBoxOverTemp)
  WatchDogReset/1 -> MATLAB Function/12(WatchDog)
